simulink model "pedestrian"  (Simulink 9.2)
settings: Solver=VariableStepAuto  StartTime=0.0  StopTime=10.0  MaxStep=1e-3  RelTol=1e-5
settings Model: Creator=jinwooro  LastModifiedBy=jinwooro
settings SolverCC: ZeroCrossAlgorithm=Adaptive
settings DataIOCC: LimitDataPoints=off  SaveFormat=Dataset  SignalLoggingSaveFormat=Dataset
settings OptimizationCC: LifeSpan=auto
settings DebuggingCC: UnderspecifiedInitializationDetection=Simplified  MergeDetectMultiDrivingBlocksExec=error  FcnCallInpInsideContextMsg=error  StateNameClashWarn=none  SFUnexpectedBacktrackingDiag=error  SFNoUnconditionalDefaultTransitionDiag=error  SFExecutionAtInitializationDiag=warning
settings HardwareCC: ProdBitPerPointer=64  ProdBitPerSizeT=64  ProdBitPerPtrDiffT=64  ProdLargestAtomicFloat=Float  ProdIntDivRoundTo=Zero  ProdEndianess=LittleEndian  ProdWordSize=64  ProdHWDeviceType=Intel->x86-64 (Windows64)
settings ModelReferenceCC: PropagateSignalLabelsOutOfModel=on
settings SFSimCC: SimUseLocalCustomCode=on
settings RTWCC: RTWUseLocalCustomCode=on
settings CodeAppCC: StateflowObjectComments=off
settings GRTTargetCC: TargetLangStandard=C99 (ISO)  GeneratePreprocessorConditionals=Use local settings  CombineOutputUpdateFcns=on  GRTInterface=off
settings ConfigComp: CovMetricSettings=dwe  CovHtmlReporting=off  CovSaveCumulativeToWorkspaceVar=off  CovSaveSingleToWorkspaceVar=off  CovExternalEMLEnable=on

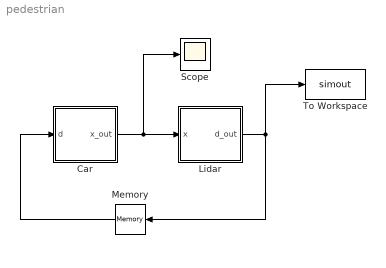
== system pedestrian ==
  Car : Stateflow chart  TreatAsAtomicUnit=on
  Lidar : Stateflow chart  TreatAsAtomicUnit=on
  Memory : Memory
  Scope : Scope
  To Workspace : ToWorkspace  VariableName=simout  SaveFormat=Timeseries  SampleTime=-1
  wires:
  Car/1(x_out) -> Scope/1, Lidar/1(x)
  Lidar/1(d_out) -> Memory/1, To Workspace/1
  Memory/1 -> Car/1(d)

== stateflow chart Lidar ==
  settings: updateMethod=CONTINUOUS
  state LidarPhysics
    du:
    d_dot = 0.2 * (x-40);
    d_out = d;
  (default) -> LidarPhysics : {
      | d = 50;
      | }
  data: d local double; x input double; d_out output double
  data d settings: updateMethod=SF_CONTINUOUS_TIME_DATA

== stateflow chart Car ==
  settings: updateMethod=CONTINUOUS
  state Moving
    du:
    x_dot = 0.2* d;
    x_out = x;
  state Stopping
    du:
    x_dot = 0;
    x_out = x;
  (default) -> Moving : {
      | x = 0;
      | }
  Moving -> Stopping : [power(d * d - 900, 1) <= 1]
  data: x local double; d input double; x_out output double
  data x settings: updateMethod=SF_CONTINUOUS_TIME_DATA
